simulink model "CAN_MultiID_Transmit_Receive_F28004x"  (R2020b)
settings: Solver=FixedStepDiscrete  StartTime=0.0  StopTime=Inf  RelTol=1e-3  EnableMultiTasking=on
undefined symbols (not defined in the file): CAN_O_IF2ARB, CANA_BASE
libraries: canmsglib x5, simulink x4, c280xlib x4, idelinklib_common x2, c2000lib x1, demo_controls x1
settings Model: ExtModeTrigDuration=8  Creator=ramalla  LastModifiedBy=swaroop
settings SolverCC: AutoInsertRateTranBlk=on
settings OptimizationCC: DefaultUnderspecifiedDataType=single  EnhancedBackFolding=on  PassReuseOutputArgsAs=Individual arguments  MaxStackSize=1024  OptimizeBlockOrder=speed  DifferentSizesBufferReuse=on  OptimizationCustomize=off  DenormalBehavior=FlushToZero  EfficientTunableParamExpr=on
settings DebuggingCC: ParameterTunabilityLossMsg=error
settings HardwareCC: ProdBitPerChar=16  ProdBitPerInt=16  ProdBitPerPointer=32  ProdBitPerSizeT=32  ProdBitPerPtrDiffT=32  ProdLargestAtomicInteger=Integer  ProdLargestAtomicFloat=None  ProdWordSize=16  ProdLongLongMode=on  ProdHWDeviceType=Texas Instruments->C2000
settings SFSimCC: MATLABDynamicMemAlloc=off
settings RTWCC: Description=Embedded Coder  SystemTargetFile=ert.tlc  HardwareBoard=TI Piccolo F280049C LaunchPad  TemplateMakefile=ert_default_tmf  Toolchain=Texas Instruments Code Composer Studio (C2000)
settings CodeAppCC: ForceParamTrailComments=on  IgnoreCustomStorageClasses=off  OperatorAnnotations=on  SimulinkDataObjDesc=on  SFDataObjDesc=on  InsertBlockDesc=on
settings ERTTargetCC: CodeReplacementLibrary=TI C28x  ExtModeTransport=3  ExtModeStaticAllocSize=5000

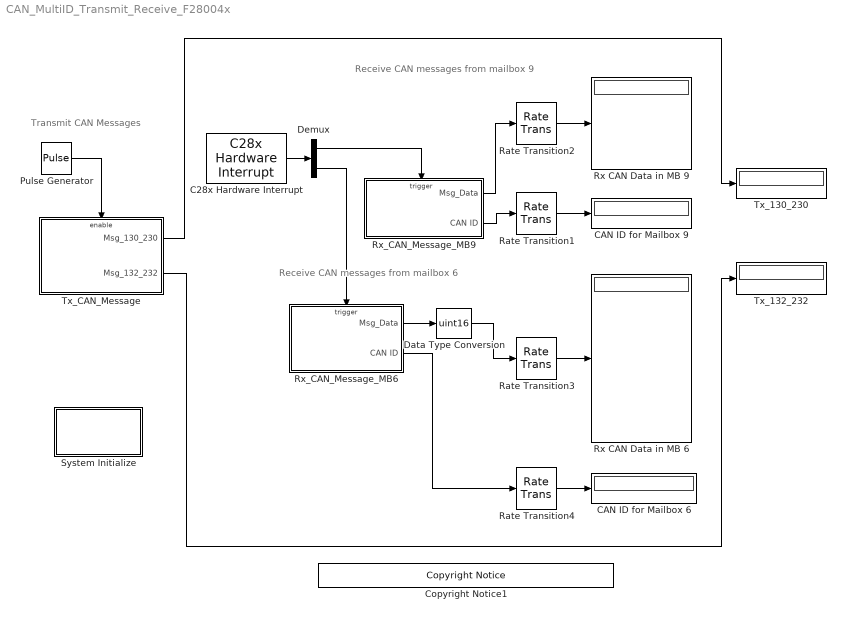
== system CAN_MultiID_Transmit_Receive_F28004x ==
  note: Receive CAN messages from mailbox 6
  note: Receive CAN messages from mailbox 9
  note: Transmit CAN Messages
  C28x Hardware Interrupt : c2000lib/Scheduling/C28x Hardware Interrupt  irqnumbers=[9 9]  pienumbers=[5 6]  irqpriorities=[0 1]  irqpreempts=[0 0]  showinput=off  dspchiptype=C280X
      settings: SourceProductBaseCode=TIC2000
  CAN ID for Mailbox 6 : Display
      settings: Format=hex (Stored Integer)
  CAN ID for Mailbox 9 : Display
      settings: Format=hex (Stored Integer)
  Copyright Notice1 : demo_controls/Copyright Notice  year=2021  prod=tic2000
      settings: SourceProductBaseCode=ME
  Data Type Conversion : DataTypeConversion  OutDataTypeStr=uint16
  Demux : Demux  Outputs=2
  Pulse Generator : DiscretePulseGenerator  Period=10  PulseWidth=3
  Rate Transition{1..4} (4 alike) : RateTransition  Integrity=off  Deterministic=off
  Rx CAN Data in MB 6 : Display
      settings: Format=decimal (Stored Integer)
  Rx CAN Data in MB 9 : Display
      settings: Format=decimal (Stored Integer)
  Rx_CAN_Message_MB6 : Subsystem  TreatAsAtomicUnit=on
  Rx_CAN_Message_MB9 : Subsystem  TreatAsAtomicUnit=on
  System Initialize : Subsystem  mask(System Initialize){ShowInLibBrowser=0}
      mask prompts: ShowInLibBrowser "Simulink:masks:CustCodeMaskParam1_MP"
      settings: CopyFcn=cccopyfcn(gcb)  OpenFcn=ccopenfcn('System Initialize Function')
      mask Help: eval('feval(''rtwprivate'',''rtwhelpview'',''rtw_sys_initialize_block'')');
      mask Display: disp('System\nInitialize');
  Tx_130_230 : Display
  Tx_132_232 : Display
  Tx_CAN_Message : Subsystem
  wires:
  Pulse Generator/1 -> Tx_CAN_Message/Enable
  Tx_CAN_Message/1(Msg_130_230) -> Tx_130_230/1
  Tx_CAN_Message/2(Msg_132_232) -> Tx_132_232/1
  C28x Hardware Interrupt/1 -> Demux/1
  Demux/2 -> Rx_CAN_Message_MB6/Trigger
  Demux/1 -> Rx_CAN_Message_MB9/Trigger
  Rx_CAN_Message_MB9/1(Msg_Data) -> Rate Transition2/1
  Rx_CAN_Message_MB9/2(CAN ID) -> Rate Transition1/1
  Rx_CAN_Message_MB6/1(Msg_Data) -> Data Type Conversion/1
  Rx_CAN_Message_MB6/2(CAN ID) -> Rate Transition4/1
  Rate Transition2/1 -> Rx CAN Data in MB 9/1
  Rate Transition1/1 -> CAN ID for Mailbox 9/1
  Rate Transition4/1 -> CAN ID for Mailbox 6/1
  Rate Transition3/1 -> Rx CAN Data in MB 6/1
  Data Type Conversion/1 -> Rate Transition3/1

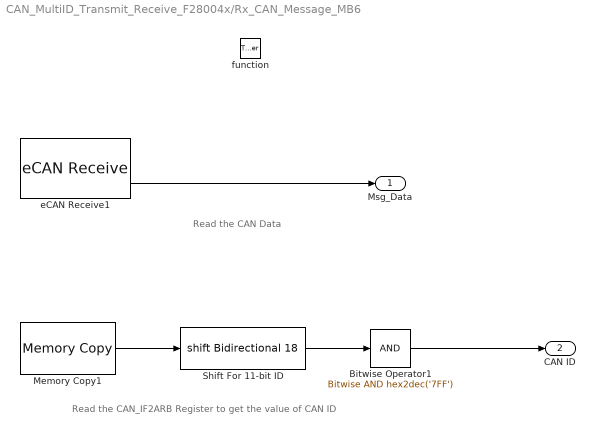
== system CAN_MultiID_Transmit_Receive_F28004x/Rx_CAN_Message_MB6 ==
  note: Read the CAN Data
  note: Read the CAN_IF2ARB Register to get the value of CAN ID
  function : TriggerPort  TriggerType=function-call  VariantControl=Variant
  Bitwise Operator1 : simulink/Logic and Bit Operations/Bitwise Operator  logicop=AND  UseBitMask=on  BitMask=hex2dec('7FF')  BitMaskRealWorld=Stored Integer
  Memory Copy1 : idelinklib_common/Memory Copy  Priority=2  copyFrom=Specified source code symbol  copyFromAddressSource=Specify via dialog  copyFromAddress=hex2dec('48108')  copyFromSrcCode=(CANA_BASE + CAN_O_IF2ARB)  dataTypeFrom=uint32  dataDimensionFrom=1  useOffsetFrom=off  offsetFromSrc=Specify via dialog  offsetFrom=0  strideFrom=1  copyTo=Output port  copyToAddressSource=Specify via dialog  copyToAddress=hex2dec('00002000')  copyToSrcCode=myVariableDst  dataTypeTo=uint32  useOffsetTo=off  offsetToSrc=Specify via dialog  offsetTo=0  strideTo=1  sampleTime=-1  useInitValue=off  initValueSrc=Specify constant value  initValue=1  initValueSrcCode=myInitValueVariable  useAsMask=off  maskOperator=bitwise AND  useTermValue=off  termValue=1  isRealtimeEnabled=off  emitCCBeforeWrite=off  CCBeforeWrite=/* Custom Code Before Write*/  emitCCAfterWrite=off  CCAfterWrite=/* Custom Code After Write*/  useDMACopy=off  enableBlockingMode=off
      settings: SourceProductBaseCode=ME
  Shift For 11-bit ID : ArithShift  BitShiftNumber=18
  eCAN Receive1 : c280xlib/eCAN Receive  Priority=1  chipFamily=C280x  useModule=eCAN_A  mailboxNo=6  messageID=108  messageType=Standard (11-bit identifier)  sampleTime=-1  dataType=uint8  initValue=0  outputMessageLength=off  outputMessageTimeStamp=off  postInterrupt=on  interruptLine=1
      settings: SourceProductName=Embedded Coder Support Package for Texas Instruments C2000 Processors
  Msg_Data : Outport
  CAN ID : Outport  Port=2
  wires:
  Bitwise Operator1/1 -> CAN ID/1
  Shift For 11-bit ID/1 -> Bitwise Operator1/1
  Memory Copy1/1 -> Shift For 11-bit ID/1
  eCAN Receive1/2 -> Msg_Data/1

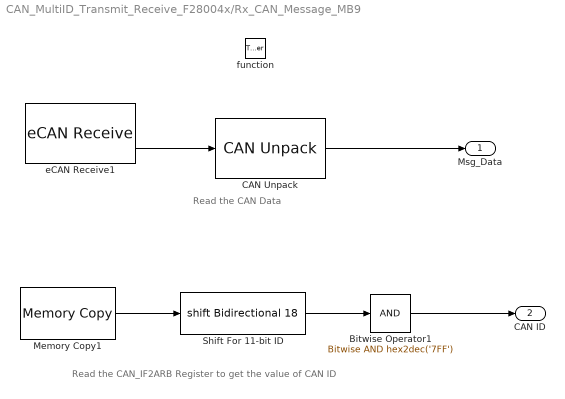
== system CAN_MultiID_Transmit_Receive_F28004x/Rx_CAN_Message_MB9 ==
  note: Read the CAN_IF2ARB Register to get the value of CAN ID
  note: Read the CAN Data
  function : TriggerPort  TriggerType=function-call  VariantControl=Variant
  Bitwise Operator1 : simulink/Logic and Bit Operations/Bitwise Operator  logicop=AND  UseBitMask=on  BitMask=hex2dec('7FF')  BitMaskRealWorld=Stored Integer
  CAN Unpack : canmsglib/CAN Unpack  MsgList=(none)  MsgName=CAN Msg  MsgIDType=Standard (11-bit identifier)  MsgIdentifier=-1  MsgLength=4  SignalInfo={}  IDPort=off  TimestampPort=off  ErrorPort=off  RemotePort=off  LengthPort=off  StatusPort=off  ApplyMinMax=off
      settings: SourceProductBaseCode=ME,XP,VN  DataFormat=raw data
  Memory Copy1 : idelinklib_common/Memory Copy  Priority=2  copyFrom=Specified source code symbol  copyFromAddressSource=Specify via dialog  copyFromAddress=hex2dec('48108')  copyFromSrcCode=(CANA_BASE + CAN_O_IF2ARB)  dataTypeFrom=uint32  dataDimensionFrom=1  useOffsetFrom=off  offsetFromSrc=Specify via dialog  offsetFrom=0  strideFrom=1  copyTo=Output port  copyToAddressSource=Specify via dialog  copyToAddress=hex2dec('00002000')  copyToSrcCode=myVariableDst  dataTypeTo=uint32  useOffsetTo=off  offsetToSrc=Specify via dialog  offsetTo=0  strideTo=1  sampleTime=-1  useInitValue=off  initValueSrc=Specify constant value  initValue=1  initValueSrcCode=myInitValueVariable  useAsMask=off  maskOperator=bitwise AND  useTermValue=off  termValue=1  isRealtimeEnabled=off  emitCCBeforeWrite=off  CCBeforeWrite=/* Custom Code Before Write*/  emitCCAfterWrite=off  CCAfterWrite=/* Custom Code After Write*/  useDMACopy=off  enableBlockingMode=off
      settings: SourceProductBaseCode=ME
  Shift For 11-bit ID : ArithShift  BitShiftNumber=18
  eCAN Receive1 : c280xlib/eCAN Receive  Priority=1  chipFamily=C280x  useModule=eCAN_A  mailboxNo=9  messageID=104  messageType=Standard (11-bit identifier)  sampleTime=-1  dataType=CAN_MESSAGE_TYPE  initValue=0  outputMessageLength=off  outputMessageTimeStamp=off  postInterrupt=on  interruptLine=0
      settings: SourceProductName=Embedded Coder Support Package for Texas Instruments C2000 Processors
  Msg_Data : Outport
  CAN ID : Outport  Port=2
  wires:
  CAN Unpack/1 -> Msg_Data/1
  Bitwise Operator1/1 -> CAN ID/1
  Memory Copy1/1 -> Shift For 11-bit ID/1
  Shift For 11-bit ID/1 -> Bitwise Operator1/1
  eCAN Receive1/2 -> CAN Unpack/1

== system CAN_MultiID_Transmit_Receive_F28004x/System Initialize ==

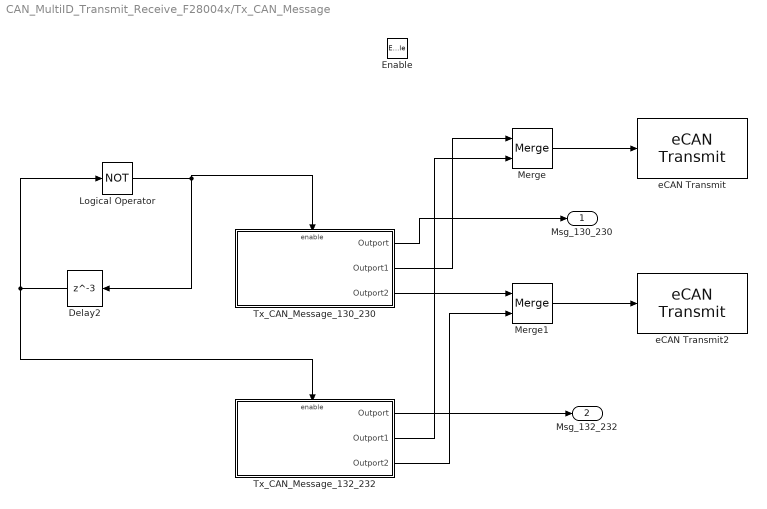
== system CAN_MultiID_Transmit_Receive_F28004x/Tx_CAN_Message ==
  Enable : EnablePort
  Delay2 : Delay  DelayLength=3  InitialCondition=0  UseCircularBuffer=on
  Logical Operator : Logic  Operator=NOT  OutDataTypeStr=boolean
  Merge : Merge
  Merge1 : Merge
  Tx_CAN_Message_130_230 : Subsystem  TreatAsAtomicUnit=on
  Tx_CAN_Message_132_232 : Subsystem  TreatAsAtomicUnit=on
  eCAN Transmit : c280xlib/eCAN Transmit  chipFamily=C280x  useModule=eCAN_A  mailboxNo=1  messageID=bin2dec('111000111')  messageType=Standard (11-bit identifier)  enableBlockingMode=on  postInterrupt=off  interruptLine=0
      settings: SourceProductName=Embedded Coder Support Package for Texas Instruments C2000 Processors
  eCAN Transmit2 : c280xlib/eCAN Transmit  chipFamily=C280x  useModule=eCAN_A  mailboxNo=2  messageID=bin2dec('111000111')  messageType=Standard (11-bit identifier)  enableBlockingMode=on  postInterrupt=off  interruptLine=0
      settings: SourceProductName=Embedded Coder Support Package for Texas Instruments C2000 Processors
  Msg_130_230 : Outport
  Msg_132_232 : Outport  Port=2
  wires:
  Logical Operator/1 -> Tx_CAN_Message_130_230/Enable, Delay2/1
  Delay2/1 -> Tx_CAN_Message_132_232/Enable, Logical Operator/1
  Tx_CAN_Message_130_230/1(Outport) -> Msg_130_230/1
  Tx_CAN_Message_132_232/1(Outport) -> Msg_132_232/1
  Tx_CAN_Message_130_230/2(Outport1) -> Merge/1
  Tx_CAN_Message_130_230/3(Outport2) -> Merge1/1
  Tx_CAN_Message_132_232/2(Outport1) -> Merge/2
  Tx_CAN_Message_132_232/3(Outport2) -> Merge1/2
  Merge/1 -> eCAN Transmit/1
  Merge1/1 -> eCAN Transmit2/1

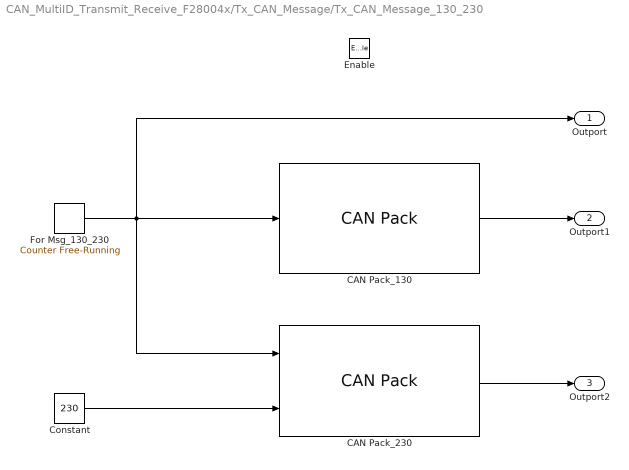
== system CAN_MultiID_Transmit_Receive_F28004x/Tx_CAN_Message/Tx_CAN_Message_130_230 ==
  Enable : EnablePort
  CAN Pack_130 : canmsglib/CAN Pack  MsgList=(none)  MsgName=CAN Msg  MsgIDType=Standard (11-bit identifier)  MsgIdentifier=hex2dec('130')  MsgLength=4  Remote=off  ApplyMinMax=off  BusOutput=off  SignalInfo={ 'Signal1', '0', '8', 'LE', 'unsigned', 'Standard', '0', '1', '0', '-Inf', 'Inf' }
      settings: SourceProductBaseCode=ME,XP,VN  DataFormat=manually specified signals
  CAN Pack_230 : canmsglib/CAN Pack  MsgList=(none)  MsgName=CAN Msg  MsgIDType=Standard (11-bit identifier)  MsgIdentifier=hex2dec('230')  MsgLength=2  Remote=off  ApplyMinMax=off  BusOutput=off  SignalInfo={ 'Signal1', '0', '8', 'LE', 'unsigned', 'Standard', '0', '1', '0', '-Inf', 'Inf'; 'Signal2', '8', '8', 'LE', 'unsigned', 'Standard', '0', '1', '0', '-Inf', 'Inf' }
      settings: SourceProductBaseCode=ME,XP,VN  DataFormat=manually specified signals
  Constant : Constant  Value=230  OutDataTypeStr=uint8
  For Msg_130_230 : simulink/Sources/Counter Free-Running  NumBits=8  tsamp=-1
  Outport : Outport
  Outport1 : Outport  Port=2
  Outport2 : Outport  Port=3
  wires:
  CAN Pack_130/1 -> Outport1/1
  For Msg_130_230/1 -> CAN Pack_230/1, Outport/1, CAN Pack_130/1
  CAN Pack_230/1 -> Outport2/1
  Constant/1 -> CAN Pack_230/2

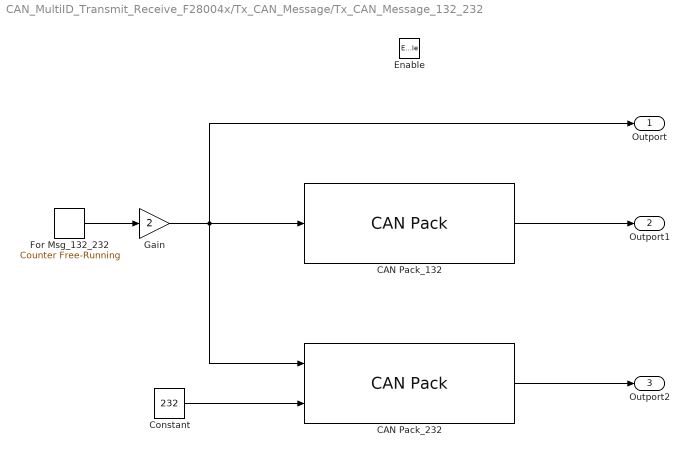
== system CAN_MultiID_Transmit_Receive_F28004x/Tx_CAN_Message/Tx_CAN_Message_132_232 ==
  Enable : EnablePort
  CAN Pack_132 : canmsglib/CAN Pack  MsgList=(none)  MsgName=CAN Msg  MsgIDType=Standard (11-bit identifier)  MsgIdentifier=hex2dec('132')  MsgLength=4  Remote=off  ApplyMinMax=off  BusOutput=off  SignalInfo={ 'Signal1', '0', '8', 'LE', 'unsigned', 'Standard', '0', '1', '0', '-Inf', 'Inf' }
      settings: SourceProductBaseCode=ME,XP,VN  DataFormat=manually specified signals
  CAN Pack_232 : canmsglib/CAN Pack  MsgList=(none)  MsgName=CAN Msg  MsgIDType=Standard (11-bit identifier)  MsgIdentifier=hex2dec('232')  MsgLength=2  Remote=off  ApplyMinMax=off  BusOutput=off  SignalInfo={ 'Signal1', '0', '8', 'LE', 'unsigned', 'Standard', '0', '1', '0', '-Inf', 'Inf'; 'Signal2', '8', '8', 'LE', 'unsigned', 'Standard', '0', '1', '0', '-Inf', 'Inf' }
      settings: SourceProductBaseCode=ME,XP,VN  DataFormat=manually specified signals
  Constant : Constant  Value=232  OutDataTypeStr=uint8
  For Msg_132_232 : simulink/Sources/Counter Free-Running  NumBits=8  tsamp=-1
  Gain : Gain  Gain=2  ParamDataTypeStr=uint8  OutDataTypeStr=uint8
  Outport : Outport
  Outport1 : Outport  Port=2
  Outport2 : Outport  Port=3
  wires:
  CAN Pack_132/1 -> Outport1/1
  For Msg_132_232/1 -> Gain/1
  Gain/1 -> CAN Pack_232/1, Outport/1, CAN Pack_132/1
  CAN Pack_232/1 -> Outport2/1
  Constant/1 -> CAN Pack_232/2
